simulink model "LQR"  (R2025b)
settings: configuration reference "code" (kept outside this file)
undefined symbols (not defined in the file or in its folder): K, TsControl
settings Model: DataDictionary=test.sldd  Creator=rpumpo  LastModifiedBy=rpumpo
settings ConfigSetRef: SourceName=code

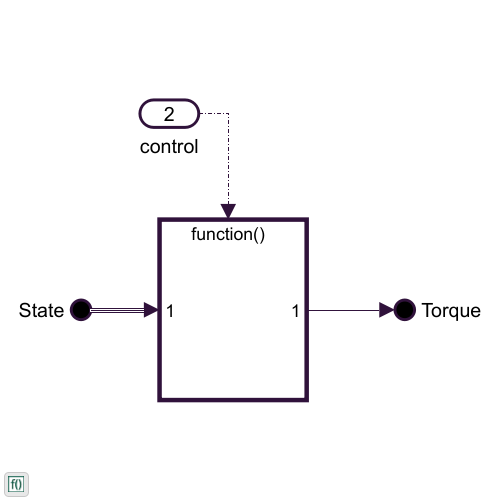
[thumbnail: Simulink's stored preview of the top-level diagram]
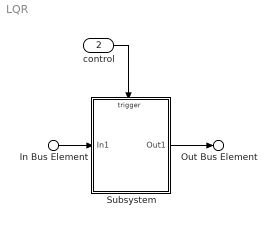
== system LQR ==
  In Bus Element : Inport  PortName=State
  control : Inport  Port=2  SampleTime=TsControl  OutputFunctionCall=on
  Subsystem : Subsystem
  Out Bus Element : Outport  PortName=Torque
  wires:
  In Bus Element/1 -> Subsystem/1(In1)
  Subsystem/1(Out1) -> Out Bus Element/1
  control/1 -> Subsystem/Trigger

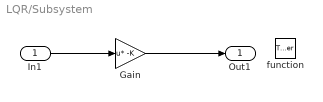
== system LQR/Subsystem ==
  In1 : Inport
  function : TriggerPort  TriggerType=function-call  VariantControl=(inherit)
  Gain : Gain  Gain=-K  Multiplication=Matrix(u*K)
  Out1 : Outport
  wires:
  In1/1 -> Gain/1
  Gain/1 -> Out1/1
